simulink model "tut04a"  (R2024b)
settings: Solver=VariableStepAuto  StartTime=0.0  StopTime=10.0  RelTol=1e-3
libraries: NSA_DEVS_LOGISTICS x8, NSA_DEVS_SINKS x6, NSA_DEVS_MATH_OPERATIONS x1, NSA_DEVS_ROUTING x1, NSA_DEVS_STATISTICS x1, NSA_DEVS_SOURCES x1
settings Model: Creator=peter  LastModifiedBy=peter

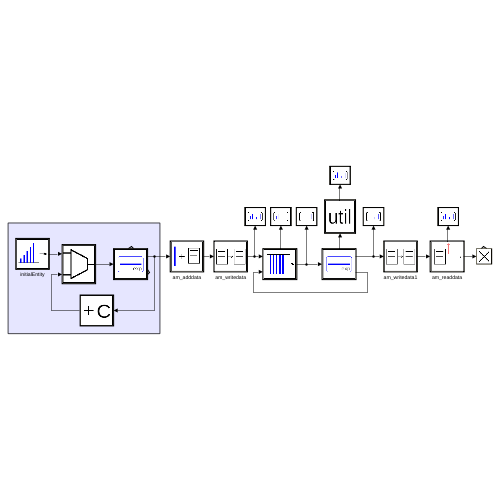
[thumbnail: Simulink's stored preview of the top-level diagram]
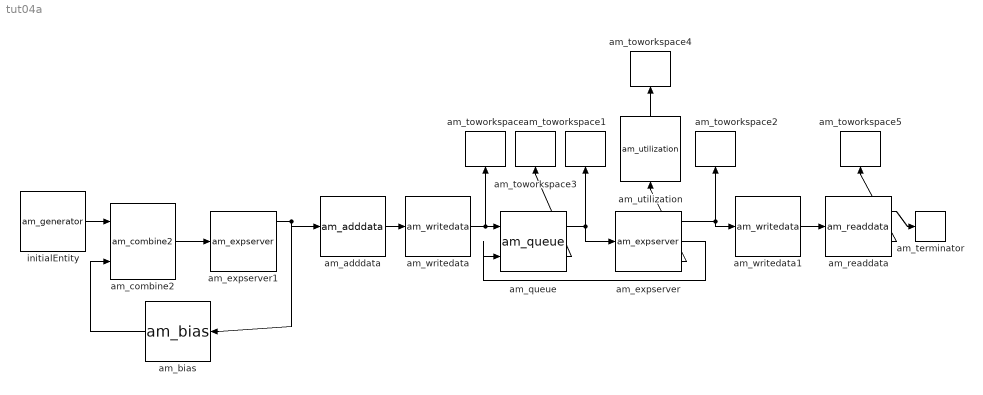
== system tut04a ==
  am_adddata : NSA_DEVS_LOGISTICS/am_adddata  fields="[\"startTime\"]"  values=[0]  numeric=[true]  infield="\"id\""  tau=[0,1]  debug=0
      settings: SourceProductName=Logistics
  am_bias : NSA_DEVS_MATH_OPERATIONS/am_bias  bias=1  tau=[0,1]  debug=0
      settings: SourceProductName=Math Operations
  am_combine2 : NSA_DEVS_ROUTING/am_combine2  tD=[0,2]  tau=[0,1]  debug=0
      settings: SourceProductName=Routing
  am_expserver : NSA_DEVS_LOGISTICS/am_expserver  tS=0.9  useSeed=false  seed=0  tau=[0,1]  debug=0
      settings: SourceProductName=Logistics
  am_expserver1 : NSA_DEVS_LOGISTICS/am_expserver  tS=1.1  useSeed=false  seed=0  tau=[0,1]  debug=0
      settings: SourceProductName=Logistics
  am_queue : NSA_DEVS_LOGISTICS/am_queue  tD=[0,2]  tau=[0,1]  debug=0
      settings: SourceProductName=Logistics
  am_readdata : NSA_DEVS_LOGISTICS/am_readdata  field="\"startTime\""  tau=[0,1]  debug=0
      settings: SourceProductName=Logistics
  am_terminator : NSA_DEVS_LOGISTICS/am_terminator  tau=[0,1]  debug=0
      settings: SourceProductName=Logistics
  am_toworkspace : NSA_DEVS_SINKS/am_toworkspace  varname="\"gen\""  t0=0  format="\"vector\""  tau=[0,5]  debug=0
      settings: SourceProductName=Sinks
  am_toworkspace1 : NSA_DEVS_SINKS/am_toworkspace  varname="\"srvIn\""  t0=0  format="\"vector\""  tau=[0,5]  debug=0
      settings: SourceProductName=Sinks
  am_toworkspace2 : NSA_DEVS_SINKS/am_toworkspace  varname="\"srvOut\""  t0=0  format="\"vector\""  tau=[0,5]  debug=0
      settings: SourceProductName=Sinks
  am_toworkspace3 : NSA_DEVS_SINKS/am_toworkspace  varname="\"qLen\""  t0=0  format="\"vector\""  tau=[0,5]  debug=0
      settings: SourceProductName=Sinks
  am_toworkspace4 : NSA_DEVS_SINKS/am_toworkspace  varname="\"sUtil\""  t0=0  format="\"vector\""  tau=[0,5]  debug=0
      settings: SourceProductName=Sinks
  am_toworkspace5 : NSA_DEVS_SINKS/am_toworkspace  varname="\"eTime\""  t0=0  format="\"vector\""  tau=[0,5]  debug=0
      settings: SourceProductName=Sinks
  am_utilization : NSA_DEVS_STATISTICS/am_utilization  tau=[0,1]  debug=0
      settings: SourceProductName=Statistics
  am_writedata : NSA_DEVS_LOGISTICS/am_writedata  inFields=[]  outField="\"startTime\""  changeFunc="\"out = get_time();\""  tau=[0,1]  debug=0
      settings: SourceProductName=Logistics
  am_writedata1 : NSA_DEVS_LOGISTICS/am_writedata  inFields="\"startTime\""  outField="\"startTime\""  changeFunc="\"out = get_time() - in(1);\""  tau=[0,1]  debug=0
      settings: SourceProductName=Logistics
  initialEntity : NSA_DEVS_SOURCES/am_generator  tG=0  n0=1  nG=1  tD=[0,2]  debug=0
      settings: SourceProductName=Sources
  wires:
  am_expserver/1 -> am_writedata1/1, am_toworkspace2/1
  am_expserver/2 -> am_queue/2
  am_queue/1 -> am_toworkspace1/1, am_expserver/1
  am_queue/2 -> am_toworkspace3/1
  am_utilization/1 -> am_toworkspace4/1
  am_expserver/3 -> am_utilization/1
  am_adddata/1 -> am_writedata/1
  am_writedata/1 -> am_queue/1, am_toworkspace/1
  am_writedata1/1 -> am_readdata/1
  am_readdata/1 -> am_terminator/1
  am_readdata/2 -> am_toworkspace5/1
  initialEntity/1 -> am_combine2/1
  am_bias/1 -> am_combine2/2
  am_combine2/1 -> am_expserver1/1
  am_expserver1/1 -> am_adddata/1, am_bias/1
